simulink model "svm"  (R2023b)
settings: Solver=VariableStepAuto  StartTime=0.0  StopTime=0.06  RelTol=1e-3
InitFcn:
  | TP=0.0002
  | Vdc=580
libraries: spsMosfetLib x6, spsSeriesRLCBranchLib x3, spsDCVoltageSourceLib x1, spsThreePhaseVIMeasurementLib x1, spsVoltageMeasurementLib x1, sps_lib x1, simulink_extras x1
settings Model: Creator=user  LastModifiedBy=user

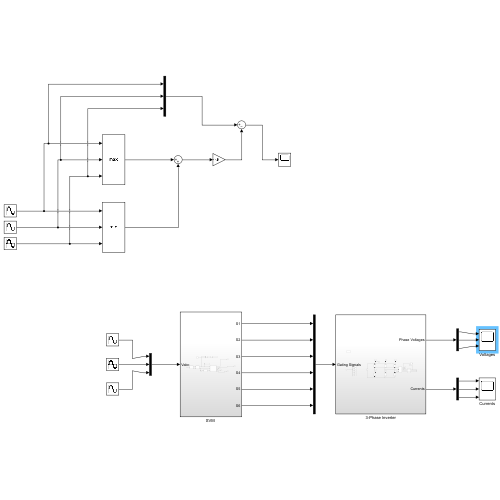
[thumbnail: Simulink's stored preview of the top-level diagram]
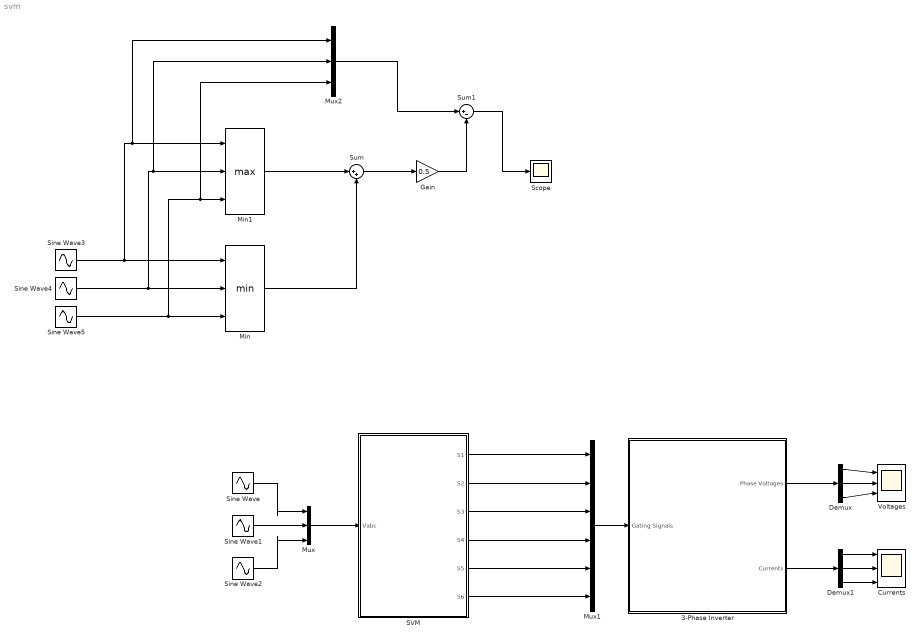
== system svm ==
  3-Phase Inverter : Subsystem
  Currents : Scope  NumInputPorts=3
  Demux : Demux  Outputs=3
  Demux1 : Demux  Outputs=3
  Gain : Gain  Gain=0.5
  Min : MinMax  Inputs=3
  Min1 : MinMax  Function=max  Inputs=3
  Mux : Mux  Inputs=3
  Mux1 : Mux  Inputs=6
  Mux2 : Mux  Inputs=3
  "SVM " : Subsystem
  Scope : Scope
  Sine Wave : Sin  Amplitude=200  Frequency=100*pi  SampleTime=1e-6
  Sine Wave1 : Sin  Amplitude=200  Frequency=100*pi  Phase=120*pi/180  SampleTime=1e-6
  Sine Wave2 : Sin  Amplitude=200  Frequency=100*pi  Phase=240*pi/180  SampleTime=1e-6
  Sine Wave3 : Sin  Amplitude=0.7*580  Frequency=100*pi  SampleTime=1e-6
  Sine Wave4 : Sin  Amplitude=0.7*580  Frequency=100*pi  Phase=120*pi/180  SampleTime=1e-6
  Sine Wave5 : Sin  Amplitude=0.7*580  Frequency=100*pi  Phase=240*pi/180  SampleTime=1e-6
  Sum : Sum  Inputs=|++
  Sum1 : Sum  Inputs=|+-
  Voltages : Scope  NumInputPorts=3
  wires:
  Sine Wave/1 -> Mux/1
  Sine Wave1/1 -> Mux/2
  Sine Wave2/1 -> Mux/3
  Mux/1 -> "SVM "/1(Vabc)
  "SVM "/1(S1) -> Mux1/1
  "SVM "/2(S2) -> Mux1/2
  "SVM "/3(S3) -> Mux1/3
  "SVM "/4(S4) -> Mux1/4
  "SVM "/5(S5) -> Mux1/5
  "SVM "/6(S6) -> Mux1/6
  Mux1/1 -> 3-Phase Inverter/1(Gating Signals)
  3-Phase Inverter/1(Phase Voltages) -> Demux/1
  Demux/3 -> Voltages/3
  Demux/1 -> Voltages/1
  Demux/2 -> Voltages/2
  Demux1/2 -> Currents/2
  Demux1/3 -> Currents/3
  Demux1/1 -> Currents/1
  3-Phase Inverter/2(Currents) -> Demux1/1
  Sine Wave3/1 -> Mux2/1, Min1/1, Min/1
  Sine Wave4/1 -> Mux2/2, Min1/2, Min/2
  Sine Wave5/1 -> Mux2/3, Min1/3, Min/3
  Min1/1 -> Sum/1
  Min/1 -> Sum/2
  Sum/1 -> Gain/1
  Mux2/1 -> Sum1/1
  Sum1/1 -> Scope/1
  Gain/1 -> Sum1/2

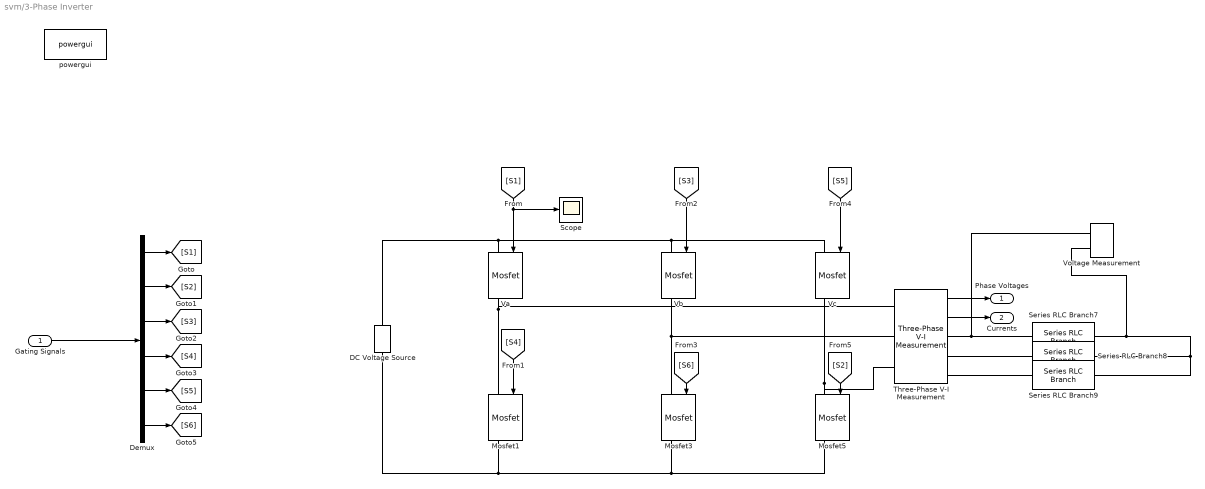
== system svm/3-Phase Inverter ==
  Gating Signals : Inport
  DC Voltage Source : spsDCVoltageSourceLib/DC Voltage Source  Amplitude=Vdc  Measurements=None
  Demux : Demux  Outputs=6
  Mosfet1 : spsMosfetLib/Mosfet  Ron=0.1  Lon=0  Rd=0.01  Vfd=0  IC=0  Rs=1e5  Cs=inf  Measurements=on
  Mosfet3 : spsMosfetLib/Mosfet  Ron=0.1  Lon=0  Rd=0.01  Vfd=0  IC=0  Rs=1e5  Cs=inf  Measurements=on
  Mosfet5 : spsMosfetLib/Mosfet  Ron=0.1  Lon=0  Rd=0.01  Vfd=0  IC=0  Rs=1e5  Cs=inf  Measurements=on
  Scope : Scope
  Series RLC Branch7 : spsSeriesRLCBranchLib/Series RLC Branch  LConnTagsString=__new0  RConnTagsString=__new0  BranchType=RL  Resistance=15  Inductance=10e-2  SetiL0=off  InitialCurrent=0  Capacitance=50e-6  Setx0=off  InitialVoltage=0  Measurements=None
  Series RLC Branch8 : spsSeriesRLCBranchLib/Series RLC Branch  LConnTagsString=__new0  RConnTagsString=__new0  BranchType=RL  Resistance=15  Inductance=10e-2  SetiL0=off  InitialCurrent=0  Capacitance=50e-6  Setx0=off  InitialVoltage=0  Measurements=None
  Series RLC Branch9 : spsSeriesRLCBranchLib/Series RLC Branch  LConnTagsString=__new0  RConnTagsString=__new0  BranchType=RL  Resistance=15  Inductance=10e-2  SetiL0=off  InitialCurrent=0  Capacitance=50e-6  Setx0=off  InitialVoltage=0  Measurements=None
  Three-Phase V-I Measurement : spsThreePhaseVIMeasurementLib/Three-Phase V-I Measurement  VoltageMeasurement=phase-to-phase  SetLabelV=off  LabelV=Vabc  Vpu=off  VpuLL=off  CurrentMeasurement=yes  SetLabelI=off  LabelI=Iabc  Ipu=off  Pbase=100e6  Vbase=500e3  OutputType=Complex  PhasorSimulation=off  PSBequivalent=0
  Va : spsMosfetLib/Mosfet  Ron=0.1  Lon=0  Rd=0.01  Vfd=0  IC=0  Rs=1e5  Cs=inf  Measurements=on
  Vb : spsMosfetLib/Mosfet  Ron=0.1  Lon=0  Rd=0.01  Vfd=0  IC=0  Rs=1e5  Cs=inf  Measurements=on
  Vc : spsMosfetLib/Mosfet  Ron=0.1  Lon=0  Rd=0.01  Vfd=0  IC=0  Rs=1e5  Cs=inf  Measurements=on
  Voltage Measurement : spsVoltageMeasurementLib/Voltage Measurement  PhasorSimulation=off  OutputType=Complex  PSBequivalent=0
  powergui : sps_lib/powergui  Priority=1  SimulationMode=Continuous  SampleTime=50e-6  frequency=60  Iterations=50  frequencyindice=0  Pbase=100e6  ErrMax=1e-4  UnitsV=kV  UnitsW=MW  buscounter=0  FunctionMessages=off  echomessages=off  EnableUseOfTLC=off  CurrentSourceSwitches=off  DisableSnubberDevices=off  DisableRonSwitches=off  DisableVfSwitches=off  DisplayEquations=off  AutomaticDiscreteSolvers=off  SolverType=Tustin/Backward Euler (TBE)  Interpol=off  ExternalGateDelay=off  methode=off  Ts=100  x0status=blocks  SPID=on  SwTol=0  HookPort=off  NonlinearTolerance=1e-4  nMaxIteration=100  ContinueOnMaxIteration=off  RestoreLinks=warning  ResistiveCurrentMeasurement=off  Frange=[0:2:500]  Ylog=off  Xlog=on  ShowGrid=off  save=off  variable=ZData  structure=0  ZoomFFT=off  StartTime=0.0  cycles=1  DisplayStyle=1  fundamental=60  FreqAxis=off  MaxFrequency=1000  frequencyindicesteady=1  RmsSteady=1  display=off
  Phase Voltages : Outport
  Currents : Outport  Port=2
  wires:
  [S6] -> Mosfet3/1
  [S2] -> Mosfet5/1
  [S3] -> Vb/1
  [S5] -> Vc/1
  [S1] -> Va/1, Scope/1
  [S4] -> Mosfet1/1
  Gating Signals/1 -> Demux/1
  Demux/1 -> [S1]
  Demux/2 -> [S2]
  Demux/3 -> [S3]
  Demux/4 -> [S4]
  Demux/5 -> [S5]
  Demux/6 -> [S6]
  Three-Phase V-I Measurement/1 -> Phase Voltages/1
  Three-Phase V-I Measurement/2 -> Currents/1
  connections:
  Mosfet1/RConn1 -- DC Voltage Source/LConn1 -- Mosfet3/RConn1 -- Mosfet5/RConn1
  Va/LConn1 -- DC Voltage Source/RConn1 -- Vc/LConn1 -- Vb/LConn1
  Vc/RConn1 -- Three-Phase V-I Measurement/LConn3 -- Mosfet5/LConn1
  Vb/RConn1 -- Mosfet3/LConn1 -- Three-Phase V-I Measurement/LConn2
  Va/RConn1 -- Mosfet1/LConn1 -- Three-Phase V-I Measurement/LConn1
  Series RLC Branch7/LConn1 -- Voltage Measurement/LConn1 -- Three-Phase V-I Measurement/RConn1
  Series RLC Branch8/LConn1 -- Three-Phase V-I Measurement/RConn2
  Series RLC Branch9/LConn1 -- Three-Phase V-I Measurement/RConn3
  Series RLC Branch9/RConn1 -- Voltage Measurement/LConn2 -- Series RLC Branch7/RConn1 -- Series RLC Branch8/RConn1

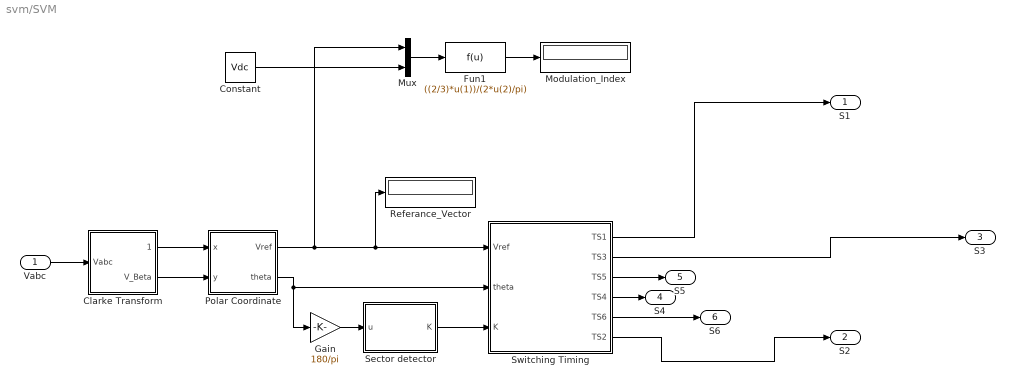
== system svm/SVM  ==
  Vabc : Inport
  Clarke Transform : Subsystem
  Constant : Constant  Value=Vdc
  Fun1 : Fcn  Expr=((2/3)*u(1))/(2*u(2)/pi)
  Gain : Gain  Gain=180/pi
  Modulation_Index : Display
  Mux : Mux  Inputs=2
  Polar Coordinate : Subsystem
  Referance_Vector : Display
  Sector detector : MATLAB Function  TreatAsAtomicUnit=on
  Switching Timing : Subsystem
  S1 : Outport
  S2 : Outport  Port=2
  S3 : Outport  Port=3
  S4 : Outport  Port=4
  S5 : Outport  Port=5
  S6 : Outport  Port=6
  wires:
  Vabc/1 -> Clarke Transform/1(Vabc)
  Clarke Transform/1(V_Alpha) -> Polar Coordinate/1(x)
  Clarke Transform/2(V_Beta) -> Polar Coordinate/2(y)
  Polar Coordinate/2(theta) -> Switching Timing/2(theta), Gain/1
  Gain/1 -> Sector detector/1(u)
  Sector detector/1(K) -> Switching Timing/3(K)
  Switching Timing/1(TS1) -> S1/1
  Mux/1 -> Fun1/1
  Constant/1 -> Mux/2
  Fun1/1 -> Modulation_Index/1
  Polar Coordinate/1(Vref) -> Mux/1, Referance_Vector/1, Switching Timing/1(Vref)
  Switching Timing/2(TS3) -> S3/1
  Switching Timing/3(TS5) -> S5/1
  Switching Timing/4(TS4) -> S4/1
  Switching Timing/5(TS6) -> S6/1
  Switching Timing/6(TS2) -> S2/1

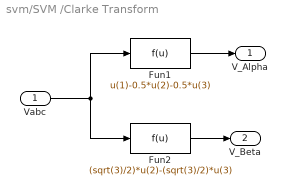
== system svm/SVM /Clarke Transform ==
  Vabc : Inport
  Fun1 : Fcn  Expr=u(1)-0.5*u(2)-0.5*u(3)
  Fun2 : Fcn  Expr=(sqrt(3)/2)*u(2)-(sqrt(3)/2)*u(3)
  V_Alpha : Outport
  V_Beta : Outport  Port=2
  wires:
  Fun1/1 -> V_Alpha/1
  Fun2/1 -> V_Beta/1
  Vabc/1 -> Fun1/1, Fun2/1

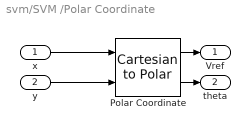
== system svm/SVM /Polar Coordinate ==
  x : Inport
  y : Inport  Port=2
  Polar Coordinate : simulink_extras/Transformations/Cartesian to Polar
  Vref : Outport
  theta : Outport  Port=2
  wires:
  y/1 -> Polar Coordinate/2
  Polar Coordinate/1 -> Vref/1
  Polar Coordinate/2 -> theta/1
  x/1 -> Polar Coordinate/1

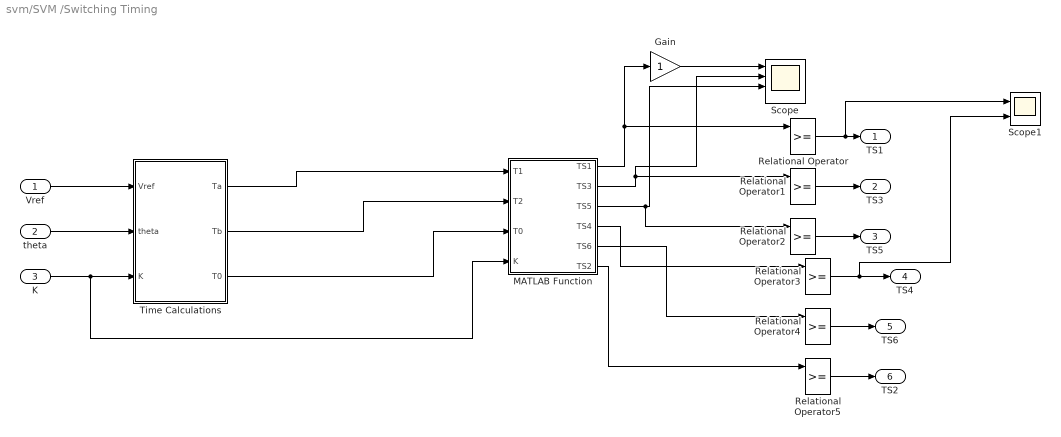
== system svm/SVM /Switching Timing ==
  Vref : Inport
  theta : Inport  Port=2
  K : Inport  Port=3
  Gain : Gain
  MATLAB Function : MATLAB Function  TreatAsAtomicUnit=on
  Relational Operator{,1..5} (6 alike) : RelationalOperator  OutDataTypeStr=boolean  RndMeth=Simplest  InputSameDT=off
  Scope : Scope  NumInputPorts=4
  Scope1 : Scope  NumInputPorts=2
  Time Calculations : Subsystem
  TS1 : Outport
  TS3 : Outport  Port=2
  TS5 : Outport  Port=3
  TS4 : Outport  Port=4
  TS6 : Outport  Port=5
  TS2 : Outport  Port=6
  wires:
  Vref/1 -> Time Calculations/1(Vref)
  theta/1 -> Time Calculations/2(theta)
  K/1 -> MATLAB Function/4(K), Time Calculations/3(K)
  Time Calculations/1(Ta) -> MATLAB Function/1(T1)
  Time Calculations/2(Tb) -> MATLAB Function/2(T2)
  Time Calculations/3(T0) -> MATLAB Function/3(T0)
  MATLAB Function/1(TS1) -> Relational Operator/1, Gain/1
  Gain/1 -> Scope/1
  Relational Operator/1 -> Scope1/1, TS1/1
  Relational Operator1/1 -> TS3/1
  MATLAB Function/2(TS3) -> Relational Operator1/1, Scope/2
  MATLAB Function/3(TS5) -> Relational Operator2/1, Scope/3
  Relational Operator2/1 -> TS5/1
  Relational Operator5/1 -> TS2/1
  MATLAB Function/6(TS2) -> Relational Operator5/1
  MATLAB Function/5(TS6) -> Relational Operator4/1
  Relational Operator4/1 -> TS6/1
  Relational Operator3/1 -> Scope1/2, TS4/1
  MATLAB Function/4(TS4) -> Relational Operator3/1

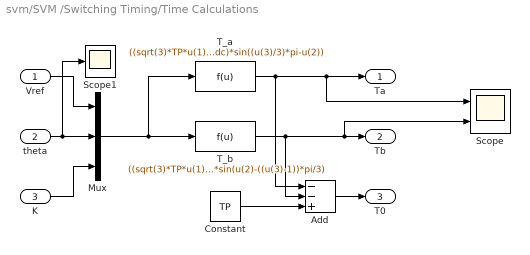
== system svm/SVM /Switching Timing/Time Calculations ==
  Vref : Inport
  theta : Inport  Port=2
  K : Inport  Port=3
  Add : Sum  Inputs=--+
  Constant : Constant  Value=TP
  Mux : Mux  Inputs=3
  Scope : Scope  NumInputPorts=2
  Scope1 : Scope
  T_a : Fcn  Expr=((sqrt(3)*TP*u(1))/Vdc)*sin((u(3)/3)*pi-u(2))
  T_b : Fcn  Expr=((sqrt(3)*TP*u(1))/Vdc)*sin(u(2)-((u(3)-1))*pi/3)
  Ta : Outport
  Tb : Outport  Port=2
  T0 : Outport  Port=3
  wires:
  Mux/1 -> T_b/1, T_a/1
  Vref/1 -> Mux/1
  K/1 -> Mux/3
  theta/1 -> Scope1/1, Mux/2
  T_a/1 -> Add/1, Scope/1, Ta/1
  T_b/1 -> Add/2, Scope/2, Tb/1
  Add/1 -> T0/1
  Constant/1 -> Add/3

== matlab function svm/SVM /Switching Timing/MATLAB Function ==
  data: TS1 output; TS3 output; TS5 output; T1 input; T2 input; T0 input; K input; TS4 output; TS6 output; TS2 output
function [TS1,TS3,TS5,TS4,TS6,TS2]= fcn(T1,T2, T0, K)
switch K

    case 1
        TS1=T1+T2+T0/2;
        TS3=T2+T0/2;
        TS5=T0/2;
        TS4=T0/2;
        TS6=T1+T0/2;
        TS2=T1+T2+T0/2;
    case 2
        TS1=T1+T0/2;
        TS3=T1+T2+T0/2;
        TS5=T0/2;
        TS4=T2+T0/2;
        TS6=T0/2;
        TS2=T1+T2+T0/2;
    case 3
        TS1=T0/2;
        TS3=T1+T2+T0/2;
        TS5=T2+T0/2;
        TS4=T1+T2+T0/2;
        TS6=T0/2;
        TS2=T1+T0/2;
    case 4
        TS1=T0/2;
        TS3=T1+T0/2;
        TS5=T1+T2+T0/2;
        TS4=T1+T2+T0/2;
        TS6=T2+T0/2;
        TS2=T0/2;
    case 5
        TS1=T2+T0/2;
        TS3=T0/2;
        TS5=T1+T2+T0/2;
        TS4=T1+T0/2;
        TS6=T1+T2+T0/2;
        TS2=T0/2;
    case 6
        TS1=T1+T2+T0/2;
        TS3=T0/2;
        TS5=T1+T0/2;
        TS4=T0/2;
        TS6=T1+T2+T0/2;
        TS2=T2+T0/2;
    otherwise
        TS1=0;
        TS3=0;
        TS5=0;
        TS2=0;
        TS4=0;
        TS6=0;
end
end

== matlab function svm/SVM /Sector detector ==
  data: u input; K output
function K = fcn(u)
Sector=0;
if(u>=0&&u<60)
    Sector=1;
elseif(u>=60&&u<120)
    Sector=2;
elseif(u>=120&&u<180)
    Sector=3;
elseif(u>=-180&&u<-120)
    Sector=4;
elseif(u>=-120&&u<-60)
    Sector=5;
elseif(u>=-60&&u<0)
    Sector=6;
end
K = Sector;
